simulink model "nonlinearAirframe"  (R2018a)
settings: Solver=ode3  StartTime=0  StopTime=50  FixedStep=Ts  RelTol=1e-3  EnableMultiTasking=on
undefined symbols (not defined in the file): e_m_X, e_m_Y, e_p_X, e_p_Y, Earth, initPosLLA, k_ac_X, k_ac_Y, k_as_X, k_as_Y, k_ra_X, k_ra_Y, k_rs_X, k_rs_Y, mass, r_m_X, r_m_Y, r_sm_X, r_sm_Y, Vehicle, WGS84
libraries: shared6dof x1, aerolibtransform2 x1
settings Model: Creator=The MathWorks, Inc.  LastModifiedBy=Ducted Fan
settings SolverCC: AutoInsertRateTranBlk=on
settings DataIOCC: SaveFormat=Array  SaveOutput=off  SignalLogging=off  DSMLogging=off  SaveTime=off
settings OptimizationCC: BlockReduction=off  DefaultParameterBehavior=Inlined  BufferReuse=off  LifeSpan=inf
settings DebuggingCC: AlgebraicLoopMsg=none  UnderspecifiedInitializationDetection=Classic  MergeDetectMultiDrivingBlocksExec=none  UnconnectedInputMsg=none  UnconnectedOutputMsg=none  UnconnectedLineMsg=none  AllowSymbolicDim=off  SFUnexpectedBacktrackingDiag=warning  SFNoUnconditionalDefaultTransitionDiag=warning  SFExecutionAtInitializationDiag=none
settings HardwareCC: ProdBitPerPointer=32  ProdBitPerSizeT=32  ProdBitPerPtrDiffT=32  ProdLargestAtomicFloat=None  ProdIntDivRoundTo=Undefined  ProdEndianess=Unspecified  ProdWordSize=32  ProdHWDeviceType=32-bit Generic
settings ModelReferenceCC: PropagateSignalLabelsOutOfModel=off
settings CodeAppCC: StateflowObjectComments=on
settings GRTTargetCC: TargetLangStandard=C89/C90 (ANSI)  GeneratePreprocessorConditionals=Disable all
settings ConfigComp: CovMetricSettings=dw  CovHtmlReporting=on  CovSaveCumulativeToWorkspaceVar=on  CovSaveSingleToWorkspaceVar=on  CovExternalEMLEnable=off  CovSFcnEnable=off

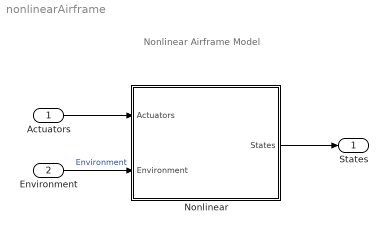
== system nonlinearAirframe ==
  note: Nonlinear Airframe Model
  Actuators : Inport  OutDataTypeStr=Bus: ActuatorsBus
  Environment : Inport  Port=2  OutDataTypeStr=Bus: EnvironmentBus  BusOutputAsStruct=on
  Nonlinear : Subsystem  TreatAsAtomicUnit=on
      mask init:
      | vehicleNonlinearVars;
      settings: MinAlgLoopOccurrences=on
  States : Outport  OutDataTypeStr=Bus: StatesBus  BusOutputAsStruct=on
  wires:
  Actuators/1 -> Nonlinear/1(Actuators)
  Environment/1 -> Nonlinear/2(Environment)  "Environment"
  Nonlinear/1(States) -> States/1

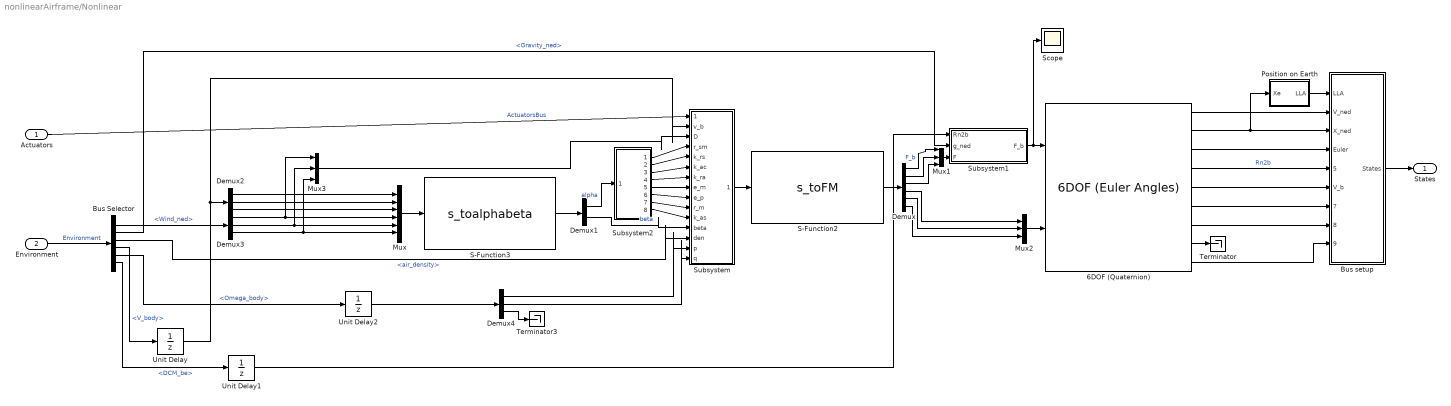
== system nonlinearAirframe/Nonlinear ==
  Actuators : Inport  OutDataTypeStr=Bus: ActuatorsBus
  Environment : Inport  Port=2  OutDataTypeStr=Bus: EnvironmentBus
  6DOF (Quaternion) : shared6dof/6DOF (Euler Angles)  units=Metric (MKS)  mtype=Fixed  rep=Euler Angles  xme_0=initPosNED  Vm_0=initVb  eul_0=initEuler  pm_0=initAngRates  mass_0=mass  mass_e=0.5  mass_f=2.0  inertia=inertia  inertia_e=eye(3)  inertia_f=2*eye(3)  k_quat=Vehicle.Nonlinear.Nonlinear.SixDOF.quatGain  vre_flag=on  abi_flag=on  aMode=aMode
      settings: SourceProductBaseCode=AE
  Bus Selector : BusSelector  OutputSignals=Wind_ned,Gravity_ned,AtmosphereBus.air_density,StatesBus.V_body,StatesBus.Omega_body,StatesBus.DCM_be
  Bus setup : Subsystem
  Demux : Demux  Outputs=6
  Demux1 : Demux  Outputs=2
  Demux2 : Demux  Outputs=3
  Demux3 : Demux  Outputs=3
  Demux4 : Demux  Outputs=3
  Mux : Mux  Inputs=6
  Mux1 : Mux  Inputs=3
  Mux2 : Mux  Inputs=3
  Mux3 : Mux  Inputs=3
  Position on Earth : Subsystem  Priority=1  TreatAsAtomicUnit=on
  S-Function2 : S-Function  FunctionName=s_toFM  SFunctionDeploymentMode=off  EnableBusSupport=off
  S-Function3 : S-Function  FunctionName=s_toalphabeta  SFunctionDeploymentMode=off  EnableBusSupport=off
  Scope : Scope
  Subsystem : Subsystem
  Subsystem1 : Subsystem
  Subsystem2 : Subsystem
  Terminator : Terminator
  Terminator3 : Terminator
  Unit Delay : UnitDelay  SampleTime=-1
  Unit Delay1 : UnitDelay  SampleTime=-1
  Unit Delay2 : UnitDelay  SampleTime=-1
  States : Outport
  wires:
  6DOF (Quaternion)/1 -> Bus setup/2(V_ned)
  6DOF (Quaternion)/2 -> Position on Earth/1(Xe), Bus setup/3(X_ned)
  6DOF (Quaternion)/3 -> Bus setup/4(Euler)
  6DOF (Quaternion)/4 -> Bus setup/5(DCM_be)  "Rn2b"
  6DOF (Quaternion)/5 -> Bus setup/6(V_b)
  6DOF (Quaternion)/6 -> Bus setup/7(Omega_b)
  6DOF (Quaternion)/7 -> Bus setup/8(dOmega_b)
  Position on Earth/1(LLA) -> Bus setup/1(LLA)
  Bus setup/1(States) -> States/1
  6DOF (Quaternion)/9 -> Bus setup/9(Accel_b)
  6DOF (Quaternion)/8 -> Terminator/1
  Actuators/1 -> Subsystem/1(Actuators)  "ActuatorsBus"
  Environment/1 -> Bus Selector/1  "Environment"
  Subsystem/1(toFM) -> S-Function2/1
  S-Function2/1 -> Demux/1
  S-Function3/1 -> Demux1/1
  Demux1/2 -> Subsystem/12(beta)  "beta"
  Mux/1 -> S-Function3/1
  Demux3/2 -> Mux3/2, Mux/5
  Demux3/1 -> Mux3/1, Mux/4
  Demux2/3 -> Mux/3
  Demux2/2 -> Mux/2
  Demux2/1 -> Mux/1
  Bus Selector/2 -> Subsystem1/2(g_ned)  "<Gravity_ned>"
  Subsystem1/1(F_b) -> Scope/1, 6DOF (Quaternion)/1
  Bus Selector/3 -> Subsystem/13(den)  "<air_density>"
  Bus Selector/1 -> Demux3/1  "<Wind_ned>"
  Demux1/1 -> Subsystem2/1(alpha)  "alpha"
  Subsystem2/1(Out1) -> Subsystem/4(r_sm)
  Subsystem2/2(Out2) -> Subsystem/5(k_rs)
  Subsystem2/3(Out3) -> Subsystem/6(k_ac)
  Subsystem2/4(Out4) -> Subsystem/7(k_ra)
  Subsystem2/5(Out5) -> Subsystem/8(e_m)
  Subsystem2/6(Out6) -> Subsystem/9(e_p)
  Subsystem2/7(Out7) -> Subsystem/10(r_m)
  Subsystem2/8(Out8) -> Subsystem/11(k_as)
  Demux/1 -> Mux1/1  "F_b"
  Demux/2 -> Mux1/2
  Demux/3 -> Mux1/3
  Mux1/1 -> Subsystem1/3(F)
  Demux/4 -> Mux2/1
  Demux/5 -> Mux2/2
  Demux/6 -> Mux2/3
  Mux2/1 -> 6DOF (Quaternion)/2
  Mux3/1 -> Subsystem/3(D)
  Demux3/3 -> Mux3/3, Mux/6
  Unit Delay/1 -> Demux2/1, Subsystem/2(v_b)
  Unit Delay1/1 -> Subsystem1/1(Rn2b)
  Unit Delay2/1 -> Demux4/1
  Demux4/1 -> Subsystem/14(p)
  Demux4/2 -> Subsystem/15(q)
  Demux4/3 -> Terminator3/1
  Bus Selector/4 -> Unit Delay/1  "<V_body>"
  Bus Selector/5 -> Unit Delay2/1  "<Omega_body>"
  Bus Selector/6 -> Unit Delay1/1  "<DCM_be>"

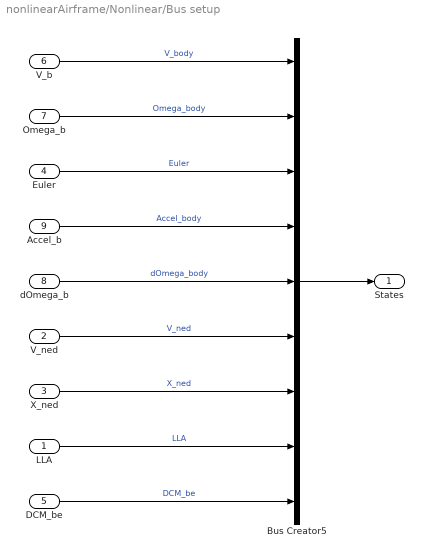
== system nonlinearAirframe/Nonlinear/Bus setup ==
  LLA : Inport  PortDimensions=3
  V_ned : Inport  Port=2  PortDimensions=3
  X_ned : Inport  Port=3  PortDimensions=3
  Euler : Inport  Port=4  PortDimensions=3
  DCM_be : Inport  Port=5  PortDimensions=[3 3]
  V_b : Inport  Port=6  PortDimensions=3
  Omega_b : Inport  Port=7  PortDimensions=3
  dOmega_b : Inport  Port=8  PortDimensions=3
  Accel_b : Inport  Port=9  PortDimensions=3
  Bus Creator5 : BusCreator  Inputs=9  OutDataTypeStr=Bus: StatesBus  NonVirtualBus=on
  States : Outport
  wires:
  Bus Creator5/1 -> States/1
  V_b/1 -> Bus Creator5/1  "V_body"
  Omega_b/1 -> Bus Creator5/2  "Omega_body"
  Euler/1 -> Bus Creator5/3  "Euler"
  X_ned/1 -> Bus Creator5/7  "X_ned"
  Accel_b/1 -> Bus Creator5/4  "Accel_body"
  LLA/1 -> Bus Creator5/8  "LLA"
  dOmega_b/1 -> Bus Creator5/5  "dOmega_body"
  DCM_be/1 -> Bus Creator5/9  "DCM_be"
  V_ned/1 -> Bus Creator5/6  "V_ned"

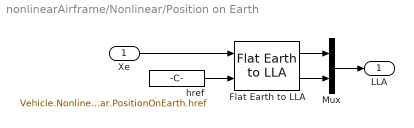
== system nonlinearAirframe/Nonlinear/Position on Earth ==
  Xe : Inport
  Flat Earth to LLA : aerolibtransform2/Flat Earth to LLA  units=Metric (MKS)  ptype=Earth (WGS84)  F=1/298.257223563  R=6378137  LL0=initPosLLA(1:2)  psi=Vehicle.Nonlinear.Nonlinear.PositionOnEarth.FlatEarthToLLA.xAxis
  Mux : Mux  Inputs=2
  href : Constant  Value=Vehicle.Nonlinear.Nonlinear.PositionOnEarth.href
  LLA : Outport
  wires:
  Mux/1 -> LLA/1
  Xe/1 -> Flat Earth to LLA/1
  Flat Earth to LLA/1 -> Mux/1
  Flat Earth to LLA/2 -> Mux/2
  href/1 -> Flat Earth to LLA/2

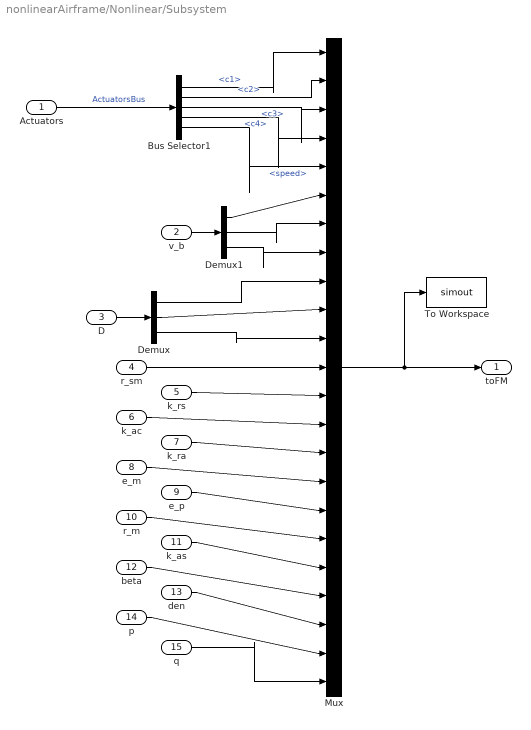
== system nonlinearAirframe/Nonlinear/Subsystem ==
  Actuators : Inport  OutDataTypeStr=Bus: ActuatorsBus
  v_b : Inport  Port=2
  D : Inport  Port=3
  r_sm : Inport  Port=4
  k_rs : Inport  Port=5
  k_ac : Inport  Port=6
  k_ra : Inport  Port=7
  e_m : Inport  Port=8
  e_p : Inport  Port=9
  r_m : Inport  Port=10
  k_as : Inport  Port=11
  beta : Inport  Port=12
  den : Inport  Port=13
  p : Inport  Port=14
  q : Inport  Port=15
  Bus Selector1 : BusSelector  OutputSignals=c1,c2,c3,c4,speed
  Demux : Demux  Outputs=3
  Demux1 : Demux  Outputs=3
  Mux : Mux  Inputs=23
  To Workspace : ToWorkspace  VariableName=simout  SaveFormat=Timeseries  SampleTime=-1
  toFM : Outport
  wires:
  Mux/1 -> To Workspace/1, toFM/1
  Actuators/1 -> Bus Selector1/1  "ActuatorsBus"
  D/1 -> Demux/1
  beta/1 -> Mux/20
  k_as/1 -> Mux/19
  r_m/1 -> Mux/18
  e_p/1 -> Mux/17
  e_m/1 -> Mux/16
  k_ra/1 -> Mux/15
  k_ac/1 -> Mux/14
  k_rs/1 -> Mux/13
  r_sm/1 -> Mux/12
  Demux/3 -> Mux/11
  Demux/2 -> Mux/10
  Demux/1 -> Mux/9
  Bus Selector1/5 -> Mux/5  "<speed>"
  Bus Selector1/4 -> Mux/4  "<c4>"
  Bus Selector1/3 -> Mux/3  "<c3>"
  Bus Selector1/2 -> Mux/2  "<c2>"
  Bus Selector1/1 -> Mux/1  "<c1>"
  den/1 -> Mux/21
  v_b/1 -> Demux1/1
  Demux1/2 -> Mux/7
  Demux1/1 -> Mux/6
  Demux1/3 -> Mux/8
  p/1 -> Mux/22
  q/1 -> Mux/23

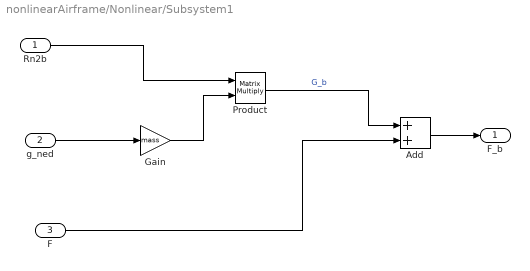
== system nonlinearAirframe/Nonlinear/Subsystem1 ==
  Rn2b : Inport
  g_ned : Inport  Port=2
  F : Inport  Port=3
  Add : Sum
  Gain : Gain  Gain=mass
  Product : Product  Multiplication=Matrix(*)
  F_b : Outport
  wires:
  g_ned/1 -> Gain/1
  Rn2b/1 -> Product/1
  Gain/1 -> Product/2
  Product/1 -> Add/1  "G_b"
  F/1 -> Add/2
  Add/1 -> F_b/1

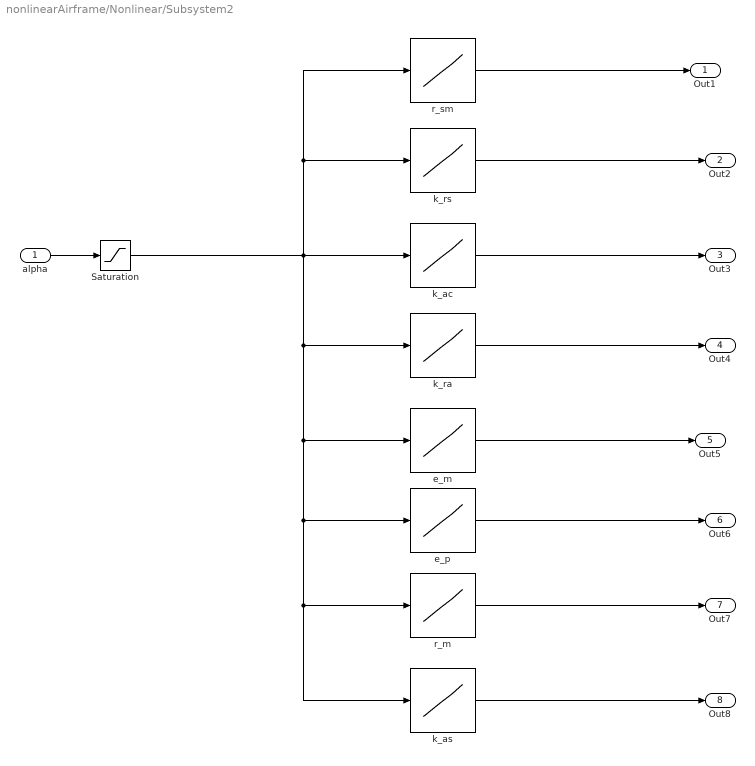
== system nonlinearAirframe/Nonlinear/Subsystem2 ==
  alpha : Inport
  Saturation : Saturate  UpperLimit=3.14159  LowerLimit=0
  e_m : Lookup_n-D  NumberOfTableDimensions=1  BreakpointsForDimension1=e_m_X  Table=e_m_Y  ExtrapMethod=Clip  DiagnosticForOutOfRangeInput=Warning  InternalRulePriority=Speed  RndMeth=Simplest  InputSameDT=on
  e_p : Lookup_n-D  NumberOfTableDimensions=1  BreakpointsForDimension1=e_p_X  Table=e_p_Y  ExtrapMethod=Clip  DiagnosticForOutOfRangeInput=Warning  InternalRulePriority=Speed  RndMeth=Simplest  InputSameDT=on
  k_ac : Lookup_n-D  NumberOfTableDimensions=1  BreakpointsForDimension1=k_ac_X  Table=k_ac_Y  ExtrapMethod=Clip  DiagnosticForOutOfRangeInput=Warning  InternalRulePriority=Speed  RndMeth=Simplest  InputSameDT=on
  k_as : Lookup_n-D  NumberOfTableDimensions=1  BreakpointsForDimension1=k_as_X  Table=k_as_Y  ExtrapMethod=Clip  DiagnosticForOutOfRangeInput=Warning  InternalRulePriority=Speed  RndMeth=Simplest  InputSameDT=on
  k_ra : Lookup_n-D  NumberOfTableDimensions=1  BreakpointsForDimension1=k_ra_X  Table=k_ra_Y  ExtrapMethod=Clip  DiagnosticForOutOfRangeInput=Warning  InternalRulePriority=Speed  RndMeth=Simplest  InputSameDT=on
  "k_rs " : Lookup_n-D  NumberOfTableDimensions=1  BreakpointsForDimension1=k_rs_X  Table=k_rs_Y  ExtrapMethod=Clip  DiagnosticForOutOfRangeInput=Warning  InternalRulePriority=Speed  RndMeth=Simplest  InputSameDT=on
  r_m : Lookup_n-D  NumberOfTableDimensions=1  BreakpointsForDimension1=r_m_X  Table=r_m_Y  ExtrapMethod=Clip  DiagnosticForOutOfRangeInput=Warning  InternalRulePriority=Speed  RndMeth=Simplest  InputSameDT=on
  r_sm : Lookup_n-D  NumberOfTableDimensions=1  BreakpointsForDimension1=r_sm_X  Table=r_sm_Y  ExtrapMethod=Clip  DiagnosticForOutOfRangeInput=Warning  InternalRulePriority=Speed  RndMeth=Simplest  InputSameDT=on
  Out1 : Outport
  Out2 : Outport  Port=2
  Out3 : Outport  Port=3
  Out4 : Outport  Port=4
  Out5 : Outport  Port=5
  Out6 : Outport  Port=6
  Out7 : Outport  Port=7
  Out8 : Outport  Port=8
  wires:
  r_sm/1 -> Out1/1
  e_p/1 -> Out6/1
  Saturation/1 -> k_as/1, r_m/1, e_p/1, e_m/1, k_ra/1, r_sm/1, "k_rs "/1, k_ac/1
  k_ac/1 -> Out3/1
  "k_rs "/1 -> Out2/1
  k_ra/1 -> Out4/1
  r_m/1 -> Out7/1
  e_m/1 -> Out5/1
  k_as/1 -> Out8/1
  alpha/1 -> Saturation/1
